simulink model "model"  (R2021a)
settings: Solver=VariableStepAuto  StartTime=0.0  StopTime=100000  RelTol=1e-3
model workspace (MATLAB code in the model file):
  | Cbs = 10;
  | Tae = 10;
libraries: slpidlib x1

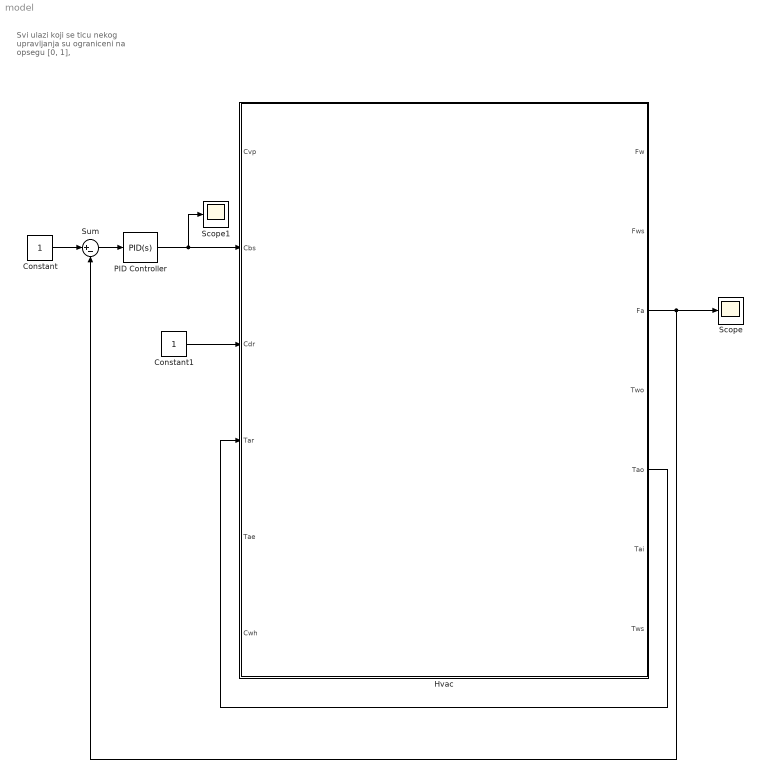
== system model ==
  note: Svi ulazi koji se ticu nekog
      | upravljanja su ograniceni na
      | opsegu [0, 1],
  Constant : Constant
  Constant1 : Constant
  Hvac : Subsystem
  PID Controller : slpidlib/PID Controller  Controller=PID  Form=Parallel  TimeDomain=Continuous-time  UseExternalTs=off  SampleTime=-1  IntegratorMethod=Forward Euler  FilterMethod=Forward Euler  ControllerParametersSource=internal  P=1  I=1  D=0  UseFilter=on  N=100  TunerSelectOption=Transfer Function Based (PID Tuner App)  InitialConditionSource=internal  InitialConditionForIntegrator=0  InitialConditionForFilter=0  DifferentiatorICPrevScaledInput=0  ExternalReset=none  TrackingMode=off  Kt=1  LimitOutput=off  SatLimitsSource=internal  UpperSaturationLimit=inf  LowerSaturationLimit=-inf  LinearizeAsGain=on  AntiWindupMode=none  Kb=1  POutMin=[]  POutMax=[]  IOutMin=[]  IOutMax=[]  DOutMin=[]  DOutMax=[]  NOutMin=[]  NOutMax=[]  SumOutMin=[]  SumOutMax=[]  SaturationOutMin=[]  SaturationOutMax=[]  PParamMin=[]  PParamMax=[]  IParamMin=[]  IParamMax=[]  DParamMin=[]  DParamMax=[]  NParamMin=[]  NParamMax=[]  KbParamMin=[]  KbParamMax=[]  KtParamMin=[]  KtParamMax=[]  KbOutMin=[]  KbOutMax=[]  KtOutMin=[]  KtOutMax=[]  IntegratorOutMin=[]  IntegratorOutMax=[]  FilterOutMin=[]  FilterOutMax=[]  SumI1OutMin=[]  SumI1OutMax=[]  SumI2OutMin=[]  SumI2OutMax=[]  SumI3OutMin=[]  SumI3OutMax=[]  SumI4OutMin=[]  SumI4OutMax=[]  SumDOutMin=[]  SumDOutMax=[]  DifferentiatorOutMin=[]  DifferentiatorOutMax=[]  FilterDiffOutCoefMin=[]  FilterDiffOutCoefMax=[]  ReciprocalOutMin=[]  ReciprocalOutMax=[]  SumDenOutMin=[]  SumDenOutMax=[]  SumNumOutMin=[]  SumNumOutMax=[]  DivideOutMin=[]  DivideOutMax=[]  UdiffTsProdOutMin=[]  UdiffTsProdOutMax=[]  NTsProdOutMin=[]  NTsProdOutMax=[]  UintegralTsProdOutMin=[]  UintegralTsProdOutMax=[]  UngainTsProdOutMin=[]  UngainTsProdOutMax=[]  IntegratorContinuousStateAttributes=''  IntegratorStateMustResolveToSignalObject=off  IntegratorRTWStateStorageClass=Auto  FilterContinuousStateAttributes=''  FilterStateMustResolveToSignalObject=off  FilterRTWStateStorageClass=Auto  ParallelPVariant=InternalParameters  IdealPVariant=Disabled  IVariant=InternalParameters  DVariant=InternalParameters  IntegratorVariant=Continuous  SatVariant=Disabled  AWVariant=Passthrough  PCopyVariant=Disabled  TRVariant=Disabled  FdbkBlocksVariant=Forward  IdealPFdbkVariant=Disabled  SatFdbkVariant=Disabled  DerivativeFilterVariant=ContFilter  NVariant=InternalParameters  NCopyVariant=Disabled  FilterICVariant=InternalICsFilter  IntegratorICVariant=InternalICs  ExternalResetVariant=Disabled  TRSumVariant=Passthrough  SumFdbkVariant=Disabled  SumVariant=Sum_PID  TsampFilterVariant=InternalTs  TsampNgainVariant=Passthrough  TsampIntegralVariant=Passthrough  ExternalSaturationOutDataTypeStr=Inherit: Same as second input
  Scope : Scope
  Scope1 : Scope
  Sum : Sum  Inputs=|+-
  wires:
  Hvac/5(Tao) -> Hvac/4(Tar)
  Sum/1 -> PID Controller/1
  Constant/1 -> Sum/1
  Hvac/3(Fa) -> Scope/1, Sum/2
  Constant1/1 -> Hvac/3(Cdr)
  PID Controller/1 -> Scope1/1, Hvac/2(Cbs)

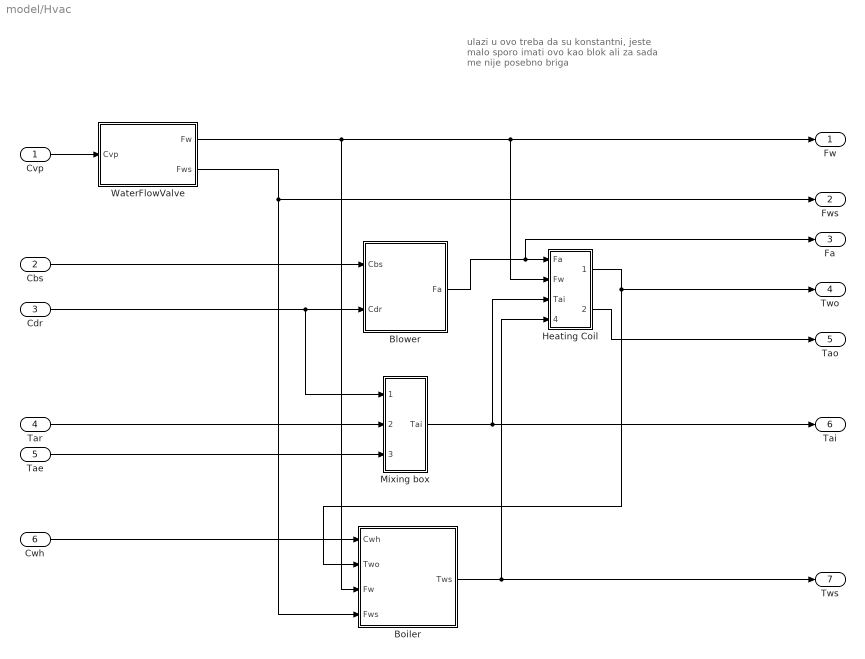
== system model/Hvac ==
  note: ulazi u ovo treba da su konstantni,
      | jeste malo sporo imati ovo kao blok
      | ali za sada me nije posebno briga
  Cvp : Inport
  Cbs : Inport  Port=2
  Cdr : Inport  Port=3
  Tar : Inport  Port=4
  Tae : Inport  Port=5
  Cwh : Inport  Port=6
  Blower : Subsystem
  Boiler : Subsystem
  Heating Coil : Subsystem
  Mixing box : Subsystem
  WaterFlowValve : Subsystem
  Fw : Outport
  Fws : Outport  Port=2
  Fa : Outport  Port=3
  Two : Outport  Port=4
  Tao : Outport  Port=5
  Tai : Outport  Port=6
  Tws : Outport  Port=7
  wires:
  Tar/1 -> Mixing box/2(Tar)
  Cvp/1 -> WaterFlowValve/1(Cvp)
  WaterFlowValve/1(Fw) -> Boiler/3(Fw), Fw/1, Heating Coil/2(Fw)
  Heating Coil/2(Tao) -> Tao/1
  WaterFlowValve/2(Fws) -> Fws/1, Boiler/4(Fws)
  Cbs/1 -> Blower/1(Cbs)
  Blower/1(Fa) -> Fa/1, Heating Coil/1(Fa)
  Boiler/1(Tws) -> Heating Coil/4(Twi), Tws/1
  Cdr/1 -> Mixing box/1(Cdr), Blower/2(Cdr)
  Heating Coil/1(Two) -> Two/1, Boiler/2(Two)
  Mixing box/1(Tai) -> Tai/1, Heating Coil/3(Tai)
  Tae/1 -> Mixing box/3(Tae)
  Cwh/1 -> Boiler/1(Cwh)

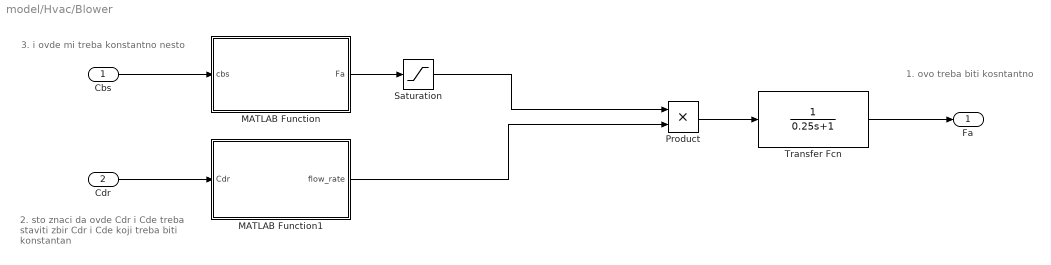
== system model/Hvac/Blower ==
  note: 3. i ovde mi treba konstantno nesto
  note: 2. sto znaci da ovde Cdr i Cde
      | treba staviti zbir Cdr i Cde koji
      | treba biti konstantan
  note: 1. ovo treba biti kosntantno
  Cbs : Inport
  Cdr : Inport  Port=2
  MATLAB Function : MATLAB Function  TreatAsAtomicUnit=on
  MATLAB Function1 : MATLAB Function  TreatAsAtomicUnit=on
  Product : Product
  Saturation : Saturate  UpperLimit=0.8058  LowerLimit=-0.04
  Transfer Fcn : TransferFcn  Denominator=[0.25 1]
  Fa : Outport
  wires:
  MATLAB Function/1(Fa) -> Saturation/1
  MATLAB Function1/1(flow_rate) -> Product/2
  Cbs/1 -> MATLAB Function/1(cbs)
  Product/1 -> Transfer Fcn/1
  Transfer Fcn/1 -> Fa/1
  Cdr/1 -> MATLAB Function1/1(Cdr)
  Saturation/1 -> Product/1

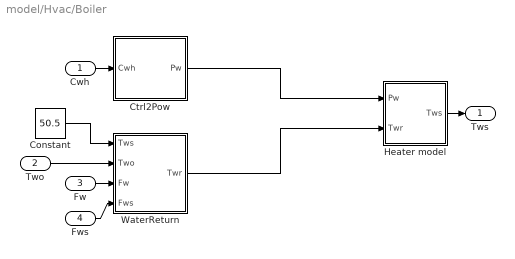
== system model/Hvac/Boiler ==
  Cwh : Inport
  Two : Inport  Port=2
  Fw : Inport  Port=3
  Fws : Inport  Port=4
  Constant : Constant  Value=50.5
  Ctrl2Pow : Subsystem
  Heater model : Subsystem
  WaterReturn : Subsystem
  Tws : Outport
  wires:
  Cwh/1 -> Ctrl2Pow/1(Cwh)
  WaterReturn/1(Twr) -> Heater model/2(Twr)
  Heater model/1(Tws) -> Tws/1
  Ctrl2Pow/1(Pw) -> Heater model/1(Pw)
  Fws/1 -> WaterReturn/4(Fws)
  Two/1 -> WaterReturn/2(Two)
  Fw/1 -> WaterReturn/3(Fw)
  Constant/1 -> WaterReturn/1(Tws)

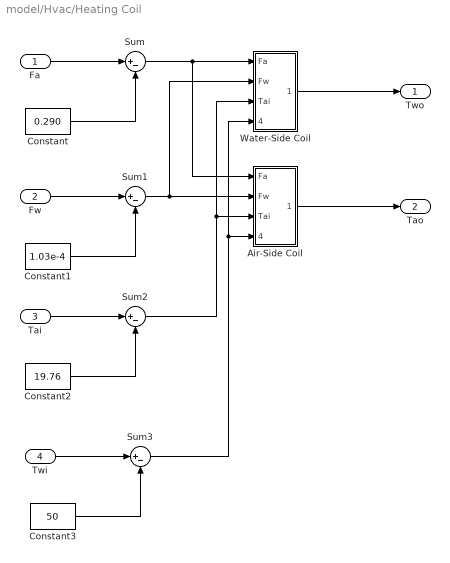
== system model/Hvac/Heating Coil ==
  Fa : Inport
  Fw : Inport  Port=2
  Tai : Inport  Port=3
  Twi : Inport  Port=4
  Air-Side Coil : Subsystem
  Constant : Constant  Value=0.290
  Constant1 : Constant  Value=1.03e-4
  Constant2 : Constant  Value=19.76
  Constant3 : Constant  Value=50
  Sum{,1..3} (4 alike) : Sum  Inputs=|+-
  Water-Side Coil : Subsystem
  Two : Outport
  Tao : Outport  Port=2
  wires:
  Twi/1 -> Sum3/1
  Tai/1 -> Sum2/1
  Constant3/1 -> Sum3/2
  Constant/1 -> Sum/2
  Air-Side Coil/1(Tao) -> Tao/1
  Constant1/1 -> Sum1/2
  Constant2/1 -> Sum2/2
  Fw/1 -> Sum1/1
  Sum2/1 -> Air-Side Coil/3(Tai), Water-Side Coil/3(Tai)
  Sum1/1 -> Air-Side Coil/2(Fw), Water-Side Coil/2(Fw)
  Water-Side Coil/1(Two) -> Two/1
  Sum/1 -> Air-Side Coil/1(Fa), Water-Side Coil/1(Fa)
  Fa/1 -> Sum/1
  Sum3/1 -> Water-Side Coil/4(Twi), Air-Side Coil/4(Twi)

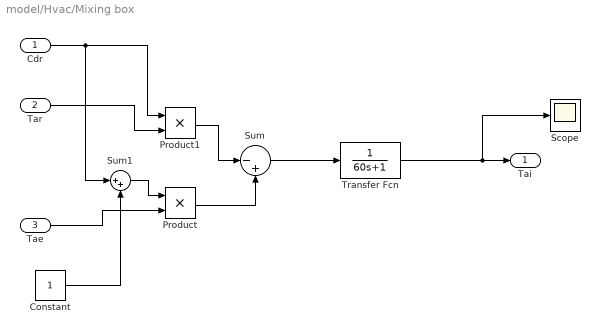
== system model/Hvac/Mixing box ==
  Cdr : Inport
  Tar : Inport  Port=2
  Tae : Inport  Port=3
  Constant : Constant
  Product : Product
  Product1 : Product
  Scope : Scope
  Sum : Sum  Inputs=|-+
  Sum1 : Sum  Inputs=|++
  Transfer Fcn : TransferFcn  Denominator=[60 1]
  Tai : Outport
  wires:
  Cdr/1 -> Sum1/1, Product1/1
  Transfer Fcn/1 -> Scope/1, Tai/1
  Tar/1 -> Product1/2
  Product/1 -> Sum/2
  Product1/1 -> Sum/1
  Sum/1 -> Transfer Fcn/1
  Tae/1 -> Product/2
  Constant/1 -> Sum1/2
  Sum1/1 -> Product/1

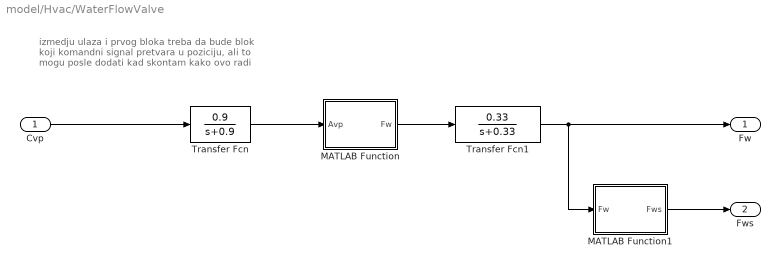
== system model/Hvac/WaterFlowValve ==
  note: izmedju ulaza i prvog bloka
      | treba da bude blok koji komandni
      | signal pretvara u poziciju, ali to mogu
      | posle dodati kad skontam kako ovo radi
  Cvp : Inport
  MATLAB Function : MATLAB Function  TreatAsAtomicUnit=on
  MATLAB Function1 : MATLAB Function  TreatAsAtomicUnit=on
  Transfer Fcn : TransferFcn  Numerator=[0.9]  Denominator=[1 0.9]
  Transfer Fcn1 : TransferFcn  Numerator=[0.33]  Denominator=[1 0.33]
  Fw : Outport
  Fws : Outport  Port=2
  wires:
  Transfer Fcn/1 -> MATLAB Function/1(Avp)
  Transfer Fcn1/1 -> Fw/1, MATLAB Function1/1(Fw)
  MATLAB Function/1(Fw) -> Transfer Fcn1/1
  Cvp/1 -> Transfer Fcn/1
  MATLAB Function1/1(Fws) -> Fws/1

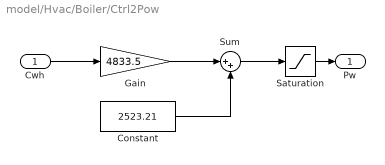
== system model/Hvac/Boiler/Ctrl2Pow ==
  Cwh : Inport
  Constant : Constant  Value=2523.21
  Gain : Gain  Gain=4833.5
  Saturation : Saturate  UpperLimit=1500  LowerLimit=0
  Sum : Sum  Inputs=|++
  Pw : Outport
  wires:
  Gain/1 -> Sum/1
  Saturation/1 -> Pw/1
  Constant/1 -> Sum/2
  Cwh/1 -> Gain/1
  Sum/1 -> Saturation/1

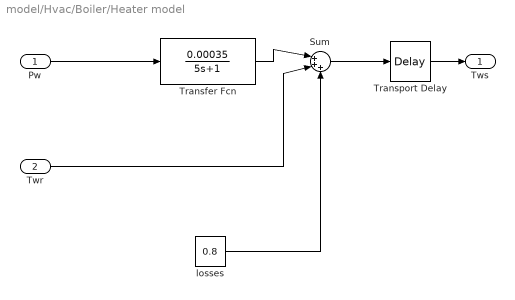
== system model/Hvac/Boiler/Heater model ==
  Pw : Inport
  Twr : Inport  Port=2
  Sum : Sum  Inputs=|+++
  Transfer Fcn : TransferFcn  Numerator=[0.00035]  Denominator=[5 1]
  Transport Delay : TransportDelay  DelayTime=12.6
  losses : Constant  Value=0.8
  Tws : Outport
  wires:
  Transfer Fcn/1 -> Sum/1
  Sum/1 -> Transport Delay/1
  Twr/1 -> Sum/2
  Transport Delay/1 -> Tws/1
  losses/1 -> Sum/3
  Pw/1 -> Transfer Fcn/1

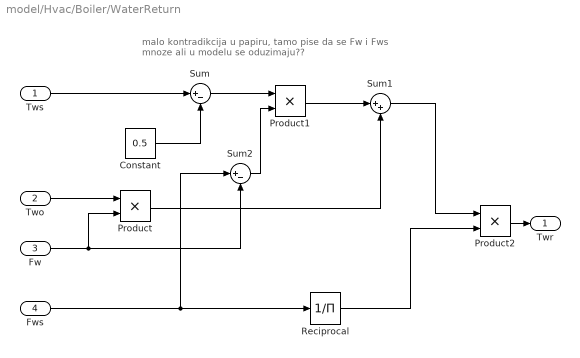
== system model/Hvac/Boiler/WaterReturn ==
  note: malo kontradikcija u papiru, tamo pise da se
      | Fw i Fws mnoze ali u modelu se oduzimaju??
  Tws : Inport
  Two : Inport  Port=2
  Fw : Inport  Port=3
  Fws : Inport  Port=4
  Constant : Constant  Value=0.5
  Product : Product
  Product1 : Product
  Product2 : Product
  Reciprocal : Product  Inputs=/
  Sum : Sum  Inputs=|+-
  Sum1 : Sum  Inputs=|++
  Sum2 : Sum  Inputs=|+-
  Twr : Outport
  wires:
  Sum1/1 -> Product2/1
  Constant/1 -> Sum/2
  Product1/1 -> Sum1/1
  Fw/1 -> Sum2/2, Product/2
  Product2/1 -> Twr/1
  Reciprocal/1 -> Product2/2
  Sum2/1 -> Product1/2
  Tws/1 -> Sum/1
  Fws/1 -> Reciprocal/1, Sum2/1
  Product/1 -> Sum1/2
  Two/1 -> Product/1
  Sum/1 -> Product1/1

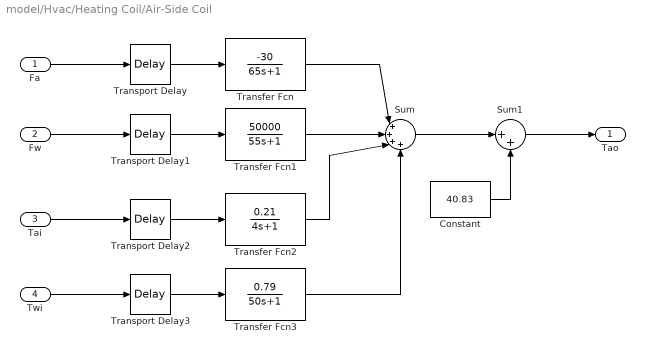
== system model/Hvac/Heating Coil/Air-Side Coil ==
  Fa : Inport
  Fw : Inport  Port=2
  Tai : Inport  Port=3
  Twi : Inport  Port=4
  Constant : Constant  Value=40.83
  Sum : Sum  Inputs=|++++
  Sum1 : Sum  Inputs=|++
  Transfer Fcn : TransferFcn  Numerator=[-30]  Denominator=[65 1]
  Transfer Fcn1 : TransferFcn  Numerator=[50000]  Denominator=[55 1]
  Transfer Fcn2 : TransferFcn  Numerator=[0.21]  Denominator=[4 1]
  Transfer Fcn3 : TransferFcn  Numerator=[0.79]  Denominator=[50 1]
  Transport Delay : TransportDelay  DelayTime=10
  Transport Delay1 : TransportDelay  DelayTime=20
  Transport Delay2 : TransportDelay  DelayTime=20
  Transport Delay3 : TransportDelay  DelayTime=20
  Tao : Outport
  wires:
  Twi/1 -> Transport Delay3/1
  Transfer Fcn3/1 -> Sum/4
  Transfer Fcn/1 -> Sum/1
  Transfer Fcn1/1 -> Sum/2
  Transport Delay/1 -> Transfer Fcn/1
  Transfer Fcn2/1 -> Sum/3
  Transport Delay2/1 -> Transfer Fcn2/1
  Constant/1 -> Sum1/2
  Fa/1 -> Transport Delay/1
  Sum/1 -> Sum1/1
  Sum1/1 -> Tao/1
  Tai/1 -> Transport Delay2/1
  Transport Delay1/1 -> Transfer Fcn1/1
  Transport Delay3/1 -> Transfer Fcn3/1
  Fw/1 -> Transport Delay1/1

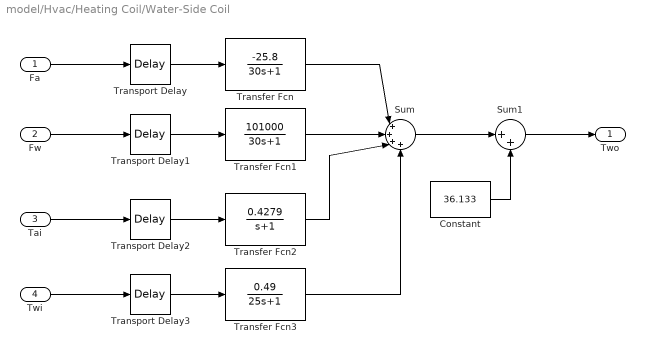
== system model/Hvac/Heating Coil/Water-Side Coil ==
  Fa : Inport
  Fw : Inport  Port=2
  Tai : Inport  Port=3
  Twi : Inport  Port=4
  Constant : Constant  Value=36.133
  Sum : Sum  Inputs=|++++
  Sum1 : Sum  Inputs=|++
  Transfer Fcn : TransferFcn  Numerator=[-25.8]  Denominator=[30 1]
  Transfer Fcn1 : TransferFcn  Numerator=[101000]  Denominator=[30 1]
  Transfer Fcn2 : TransferFcn  Numerator=[0.4279]  Denominator=[1 1]
  Transfer Fcn3 : TransferFcn  Numerator=[0.49]  Denominator=[25 1]
  Transport Delay : TransportDelay  DelayTime=15
  Transport Delay1 : TransportDelay  DelayTime=10
  Transport Delay2 : TransportDelay  DelayTime=10
  Transport Delay3 : TransportDelay  DelayTime=40
  Two : Outport
  wires:
  Twi/1 -> Transport Delay3/1
  Transfer Fcn3/1 -> Sum/4
  Transfer Fcn/1 -> Sum/1
  Transfer Fcn1/1 -> Sum/2
  Transport Delay/1 -> Transfer Fcn/1
  Transfer Fcn2/1 -> Sum/3
  Transport Delay2/1 -> Transfer Fcn2/1
  Constant/1 -> Sum1/2
  Fa/1 -> Transport Delay/1
  Sum/1 -> Sum1/1
  Sum1/1 -> Two/1
  Tai/1 -> Transport Delay2/1
  Transport Delay1/1 -> Transfer Fcn1/1
  Transport Delay3/1 -> Transfer Fcn3/1
  Fw/1 -> Transport Delay1/1

== matlab function model/Hvac/Blower/MATLAB Function ==
  data: Fa output; cbs input
function Fa = cbs2Fa(cbs)
    % Blower speed control to airflow
    Fa = 1.23e-8 * cbs^4 - 3.93e-6 * cbs^3 ...
        + 10e-4 * cbs^2 - 2.32e-3 * cbs - 1.7e-2;

== matlab function model/Hvac/WaterFlowValve/MATLAB Function ==
  data: Avp input; Fw output
function Fw = Avp2Fw(Avp)
    Fw = -4.9e-12 * Avp^4 + 1.3e-9 * Avp^3 - 6.9e-8 * Avp^2 ...
        + 4.5e-6 * Avp - 7.8e-8;

== matlab function model/Hvac/WaterFlowValve/MATLAB Function1 ==
  data: Fw input; Fws output
function Fws = Fw2Fws(Fw)
    Fws = -240966 * Fw^3 + 888 * Fw^2 - 0.53915 * Fw + 0.00063;

== matlab function model/Hvac/Blower/MATLAB Function1 ==
  data: Cdr input; flow_rate output
function flow_rate = adjFa(Cdr)
    flow_rate = -0.0233*Cdr^3 - 0.0287 * Cdr^2 + 0.0119*Cdr + 0.933;
